simulink model "RefModel_Task"  (R2020a)
settings: Solver=ode1  StartTime=0.0  StopTime=10.0  FixedStep=Ts_Task.Ts_base  RelTol=1e-3
undefined symbols (not defined in the file or in its folder): groundspeedCmd, heightCmd, rollCmd
(part 5 of 5)

== matlab function RefModel_Task/Data Display/MATLAB Function ==
  data: u input; u output
function u = fcn(u)
for i = 1:3
    if u(i) == 0
        u(i) = nan;
    end
end

== matlab function RefModel_Task/Data Display/MATLAB Function1 ==
  data: u input; u output
function u = fcn(u)
for i = 1:3
    if u(i) == 0
        u(i) = nan;
    end
end

== matlab function RefModel_Task/Data Display/debug logDataBuffer ==
  data: logDataOut input; u input Bus: BUS_TASK_SingleLog size=TASK_PARAM_V1000.logDataBufferSize; y_out output Enum: ENUM_RTInfo_Task; TaskParam input Bus: BUS_TASK_PATH_AlgoParam size=1; y_buffer output Enum: ENUM_RTInfo_Task size=TASK_PARAM_V1000.logDataBufferSize
function [y_out,y_buffer] = fcn(logDataOut, u, TaskParam)
y_buffer = ENUM_RTInfo_Task(zeros(32,1));
y_out = ENUM_RTInfo_Task(zeros(3,1));
for i = 1:TaskParam.logDataBufferSize
    y_buffer(i) = u(i).message;
end
for i = 1:TaskParam.logDataOutSize
    y_out(i) = logDataOut(i).message;
end

== matlab function RefModel_Task/Cmd Protect/Subsystem1/MATLAB Function ==
  data: u input; y output; maxRoll input
function y = fcn(u, maxRoll)
if u > maxRoll
    y = maxRoll;
elseif u < -maxRoll
    y = -maxRoll;
else
    y = u;
end
